simulink model "dcmg"  (R2020a)
settings: Solver=VariableStepAuto  StartTime=0.0  StopTime=Inf  FixedStep=50e-6  RelTol=1e-3
PostLoadFcn:
  | , if any(exist('dsrtsu_mdlpostloadfcn', 'file') ~= 0), dsrtsu_mdlpostloadfcn('Execute', bdroot); end,
InitFcn:
  | , if any(exist('rtifpga_mdlclblib', 'file') ~= 0), rtifpga_mdlclblib('Init', bdroot); end,
model workspace (MAT data in the model file):
  FPGA_dcmg_1_Register_1_1_1_write = Simulink.Signal
  FPGA_dcmg_1_Register_1_1_1_write.Description = 'RTIFPGA'
  FPGA_dcmg_1_Register_1_1_1_write.DataType = 'double'
  FPGA_dcmg_1_Register_1_1_1_write.Dimensions = '1'
  FPGA_dcmg_1_Register_1_1_1_write.DimensionsMode = 'auto'
  FPGA_dcmg_1_Register_1_1_1_write.Complexity = 'auto'
  FPGA_dcmg_1_Register_1_1_1_write.SampleTime = -1
  FPGA_dcmg_1_Register_1_1_1_write.SamplingMode = 'auto'
  FPGA_dcmg_1_Register_2_1_1_write = Simulink.Signal
  FPGA_dcmg_1_Register_2_1_1_write.Description = 'RTIFPGA'
  FPGA_dcmg_1_Register_2_1_1_write.DataType = 'double'
  FPGA_dcmg_1_Register_2_1_1_write.Dimensions = '1'
  FPGA_dcmg_1_Register_2_1_1_write.DimensionsMode = 'auto'
  FPGA_dcmg_1_Register_2_1_1_write.Complexity = 'auto'
  FPGA_dcmg_1_Register_2_1_1_write.SampleTime = -1
  FPGA_dcmg_1_Register_2_1_1_write.SamplingMode = 'auto'
  FPGA_dcmg_1_Register_3_1_1_write = Simulink.Signal
  FPGA_dcmg_1_Register_3_1_1_write.Description = 'RTIFPGA'
  FPGA_dcmg_1_Register_3_1_1_write.DataType = 'double'
  FPGA_dcmg_1_Register_3_1_1_write.Dimensions = '1'
  FPGA_dcmg_1_Register_3_1_1_write.DimensionsMode = 'auto'
  FPGA_dcmg_1_Register_3_1_1_write.Complexity = 'auto'
  FPGA_dcmg_1_Register_3_1_1_write.SampleTime = -1
  FPGA_dcmg_1_Register_3_1_1_write.SamplingMode = 'auto'
  FPGA_dcmg_1_Register_4_1_1_write = Simulink.Signal
  FPGA_dcmg_1_Register_4_1_1_write.Description = 'RTIFPGA'
  FPGA_dcmg_1_Register_4_1_1_write.DataType = 'double'
  FPGA_dcmg_1_Register_4_1_1_write.Dimensions = '1'
  FPGA_dcmg_1_Register_4_1_1_write.DimensionsMode = 'auto'
  FPGA_dcmg_1_Register_4_1_1_write.Complexity = 'auto'
  FPGA_dcmg_1_Register_4_1_1_write.SampleTime = -1
  FPGA_dcmg_1_Register_4_1_1_write.SamplingMode = 'auto'
  FPGA_dcmg_1_Register_5_1_1_write = Simulink.Signal
  FPGA_dcmg_1_Register_5_1_1_write.Description = 'RTIFPGA'
  FPGA_dcmg_1_Register_5_1_1_write.DataType = 'double'
  FPGA_dcmg_1_Register_5_1_1_write.Dimensions = '1'
  FPGA_dcmg_1_Register_5_1_1_write.DimensionsMode = 'auto'
  FPGA_dcmg_1_Register_5_1_1_write.Complexity = 'auto'
  FPGA_dcmg_1_Register_5_1_1_write.SampleTime = -1
  FPGA_dcmg_1_Register_5_1_1_write.SamplingMode = 'auto'
values from neighbouring files (symbols this model uses):
  den = [1, zeros(1,499)]    [params.m]
  fixedgain_i = 10*1000/(3*100)    (= 33.3333333333)    [param.m]    (also in params.m)
  fixedgain_ibat = 10*1000/(3*100)    (= 33.3333333333)    [params.m]
  fixedgain_ipv = 10*1000/(3*100)    (= 33.3333333333)    [params.m]
  fixedgain_v = 10*22000/(3*100*2.5)    (= 293.333333333)    [params.m]
  fixedgain_vdc = 10*22000/(3*100*2.5)    (= 293.333333333)    [param.m]    (also in params.m = 586.666666667)
  fixedgain_vpv = 10*10000/(3*100*2.5)    (= 133.333333333)    [params.m]
  gain_iavsi = 1    [params.m]
  gain_ibat = 1    [params.m]
  gain_ibvsi = 1    [params.m]
  gain_icvsi = 1    [params.m]
  gain_ioavsi = 1    [params.m]
  gain_iobvsi = 1    [params.m]
  gain_ipv = 1    [params.m]
  gain_sinwave = 0.3    [params.m]
  gain_vavsi = 1    [params.m]
  gain_vbvsi = 1    [params.m]
  gain_vcvsi = 1    [params.m]
  gain_vdc = 1    [param.m]    (also in params.m)
  gain_vpv = 1    [params.m]
  N = 10    [param.m]    (also in params.m = 100)
  num = 1/500*ones(1,500)    [params.m]
  offset_iavsi = 0.2    [params.m]
  offset_ibat = 0    [params.m]
  offset_ibvsi = 0.2    [params.m]
  offset_icvsi = 0.2    [params.m]
  offset_ioavsi = 0    [params.m]
  offset_iobvsi = 0    [params.m]
  offset_ipv = 0    [params.m]
  offset_vavsi = 0    [params.m]
  offset_vbvsi = 0    [params.m]
  offset_vcvsi = 0    [params.m]
  offset_vdc = 1.5    [param.m]    (also in params.m = 0)
  offset_vpv = 0    [params.m]
  v_dc_ref = 40    [param.m]    (also in params.m = 24)
libraries: xbsIndex_r4 x258, rti1202lib_adc_class1 x10, rtiproclib x9, simulink x5, rti1202lib_adc_class2 x2, rtifpgainterfacelib x1
(part 1 of 7)
Description:
  | Standard RTI1202 template.
  | Supported MATLAB version:  R2020a.
settings Model: Tag=RTI1202  DSRTSU_INTERNAL_RTI_VER=570  DSRTSU_INTERNAL_RTI_TYPE=rti1202  RTICANMMDATA=struct('GeneralSetupData',struct('modelroot','D:\MarcosGomez\DCMG','generalsettings',struct('filesettings',struct('destfolder',struct('Name','RTICANMM_FILES','Check',1),'buildfolder',struct('Name','.','Check',1),'AbsDestfolder',struct('Name','D:\MarcosGomez\DCMG\RTICANMM_FILES'),'AbsBuildfolder',struct('Name','D:\MarcosGomez\DCMG'))),'options',struct('addpaths',1,'rmpaths',1,'addtrcexclusion',true,'cannavigator',struct('checkmonitoring',0),'show_usrtrc',0,'use_usrtrc',0),'advanced',struct('options',ones(1,100)),'MPSetup',{{}},'RTI',struct('Type','RTI1202','Ver','7.15','Date','02-Nov-2020'),'modelname','dcmg','block','dcmg'))  DSRTSU_INTERNAL_RTIFPGA=170  OrderedModelArguments=off  Creator=dspace  LastModifiedBy=dspace
settings DataIOCC: ReturnWorkspaceOutputs=off
settings OptimizationCC: BlockReduction=off  OptimizeBlockIOStorage=off  BufferReuse=off  GlobalBufferReuse=off  ExpressionFolding=off  LocalBlockOutputs=off  OptimizeDataStoreBuffers=off  BusAssignmentInplaceUpdate=off
settings DebuggingCC: PregeneratedLibrarySubsystemCodeDiagnostic=none  ArithmeticOperatorsInVariantConditions=warning
settings HardwareCC: ProdBitPerPointer=32  ProdBitPerSizeT=32  ProdBitPerPtrDiffT=32  ProdLargestAtomicInteger=Integer  ProdEndianess=BigEndian  ProdWordSize=32  ProdLongLongMode=on  ProdHWDeviceType=Custom Processor->Custom  TargetIntDivRoundTo=Zero  TargetEndianess=BigEndian  TargetHWDeviceType=Custom Processor->Custom
settings ModelReferenceCC: EnableParallelModelReferenceBuilds=on  ParallelModelReferenceMATLABWorkerInit=Load Top Model
settings SFSimCC: SimUseLocalCustomCode=off  MATLABDynamicMemAlloc=off  CustomCodeUndefinedFunction=UseInterfaceOnly
settings RTWCC: Description=dSPACE DS1202 Hardware Platform  SystemTargetFile=rti1202.tlc  MakeCommand=make_rti  TemplateMakefile=rti1202.tmf  RTWUseLocalCustomCode=off
settings CodeAppCC: StateflowObjectComments=on
settings STFCustomTargetCC: ParMdlRefBuildCompliant=on  SystemTargetFile=rti1202.tlc
settings GRTTargetCC: TargetLangStandard=C89/C90 (ANSI)  CompOptLevelCompliant=off  ConcurrentExecutionCompliant=off  CombineOutputUpdateFcns=off  MatFileLogging=off  CPPClassGenCompliant=off  UseToolchainInfoCompliant=off
settings ConfigComp: CovMetricSettings=dswe

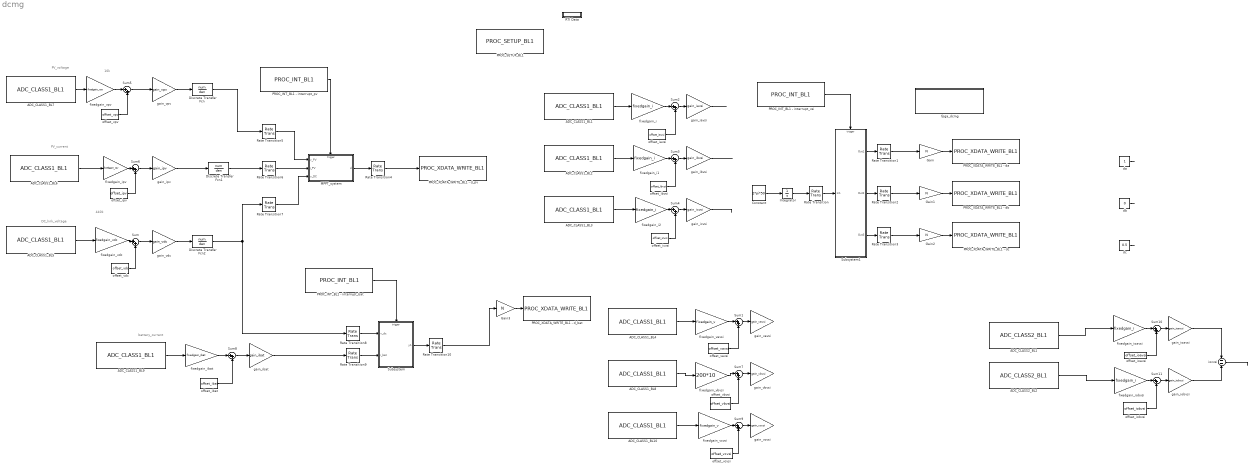
== system dcmg ==
  note: PV_voltage
  note: 10k
  note: 440k
  note: DC_link_voltage
  note: PV_current
  note: battery_current
  ADC_CLASS1_BL1 : rti1202lib_adc_class1/ADC_CLASS1_BL1  DSProperties=struct('RTI',struct('Version',uint32(1),'BlockType',struct('isSLSource',uint8(1),'isSLSink',uint8(1),'isHWSource',uint8(0),'isHWSink',uint8(1),'isSetup',uint8(0),'isInline',uint8(1),'isNonInline',uint8(0),'isInterrupt',uint8(0),'isChannelwise',uint8(1)),'IOBoardType',{{'DS120X','STD','ADCC1'}},'UnitType','ADC','Identifier','ADC','DialogType','ML','BlockSet','NONE','SlaveProcessor','NONE'))  RTIBlockInterface=struct('InputPortsActive',0,'InputPortsWidth',int32(1),'InputPortsDataType',{{'SS_BOOLEAN'}},'InputPortsName',{{'Continue'}},'OutputPortsActive',[1 0],'OutputPortsWidth',int32([1 1]),'OutputPortsDataType',{{'SS_DOUBLE','SS_INT16'}},'OutputPortsName',{{'ADC','Status'}},'DialogFcn','rti120xstdadcc1adcgui','SampleTime',{{-1}},'InitLevel',3,'IconTransparency','on','BlockDisplay',{{['ADC CL1\nChannel: 15'],'center'}},'BlockName',struct('Token',{{'ADC_CLASS1_BL1'}}))  RTIBlockParameters=struct('ReadMode',{{1,'OFF',[1 2]}},'ChannelNo',{{15,'OFF',[]}},'ConversionMode',{{1,'OFF',[1 2]}},'TriggerSource',{{1,'OFF',[1 2]}},'TriggerLineIn',{{1,'OFF',[1 16]}},'SampleMode',{{1,'OFF',[1 2]}},'BurstTriggerSource',{{1,'OFF',[1 2]}},'BurstTriggerLine',{{1,'OFF',[1 16]}},'ConvTriggerSource',{{3,'OFF',[1 3]}},'ConvTriggerLine',{{1,'OFF',[1 16]}},'ConvPeriod',{{'100e-6','OFF',[1e-6 1.34]}},'ConvPeriodCheck',{{0,'OFF',[]}},'BurstSize',{{'10','OFF',[]}},'BurstSizeCheck',{{0,'OFF',[]}},'DataSetOffset',{{'0','OFF',[]}},'DataSetOffsetCheck',{{0,'OFF',[]}},'DataSetLength',{{'1','OFF',[]}},'DataSetLengthCheck',{{0,'OFF',[]}},'EnableTriggerEvent',{{0,'OFF',[0 1]}},'TriggerMode',{{2,'OFF',[1 3]}},'TriggerLineOut',{{1,'OFF',[1 16]}},'ADCSWStartEnable',{{0,'OFF',[0 1]}},'SampleTime',{{'-1','OFF',[-1 inf]}},'SampleTimeCheck',{{1,'OFF',[]}},'StatusPortEnable',{{0,'OFF',[0 1]}},'TLCFileName',{{'rti120xadc_c1_adc','OFF',[]}})  RTISFcnParameters=struct('ReadMode','int16','ChannelNo','int16','ConversionMode','int16','TriggerSource','int16','TriggerLineIn','int16','SampleMode','int16','BurstTriggerSource','int16','BurstTriggerLine','int16','ConvTriggerSource','int16','ConvTriggerLine','int16','ConvPeriod','double','BurstSize','int16','DataSetOffset','int16','DataSetLength','int16','EnableTriggerEvent','int16','TriggerMode','int16','TriggerLineOut','int16','ADCSWStartEnable','int16','SampleTime','double','StatusPortEnable','int16','TLCFileName','char')  RTIBlockParaDefault=struct('ReadMode',1,'ChannelNo',1,'ConversionMode',1,'TriggerSource',1,'TriggerLineIn',1,'SampleMode',1,'BurstTriggerSource',1,'BurstTriggerLine',1,'ConvTriggerSource',3,'ConvTriggerLine',1,'ConvPeriod',0.0001,'ConvPeriodCheck',0,'BurstSize',10,'BurstSizeCheck',0,'DataSetOffset',0,'DataSetOffsetCheck',0,'DataSetLength',1,'DataSetLengthCheck',0,'EnableTriggerEvent',0,'TriggerMode',2,'TriggerLineOut',1,'ADCSWStartEnable',0,'SampleTime',-1,'SampleTimeCheck',1,'StatusPortEnable',0,'TLCFileName','rti120xadc_c1_adc')
  ADC_CLASS1_BL10 : rti1202lib_adc_class1/ADC_CLASS1_BL1  DSProperties=struct('RTI',struct('Version',uint32(1),'BlockType',struct('isSLSource',uint8(1),'isSLSink',uint8(1),'isHWSource',uint8(0),'isHWSink',uint8(1),'isSetup',uint8(0),'isInline',uint8(1),'isNonInline',uint8(0),'isInterrupt',uint8(0),'isChannelwise',uint8(1)),'IOBoardType',{{'DS120X','STD','ADCC1'}},'UnitType','ADC','Identifier','ADC','DialogType','ML','BlockSet','NONE','SlaveProcessor','NONE'))  RTIBlockInterface=struct('InputPortsActive',0,'InputPortsWidth',int32(1),'InputPortsDataType',{{'SS_BOOLEAN'}},'InputPortsName',{{'Continue'}},'OutputPortsActive',[1 0],'OutputPortsWidth',int32([1 1]),'OutputPortsDataType',{{'SS_DOUBLE','SS_INT16'}},'OutputPortsName',{{'ADC','Status'}},'DialogFcn','rti120xstdadcc1adcgui','SampleTime',{{-1}},'InitLevel',3,'IconTransparency','on','BlockDisplay',{{['ADC CL1\nChannel: 20'],'center'}},'BlockName',struct('Token',{{'ADC_CLASS1_BL1'}}))  RTIBlockParameters=struct('ReadMode',{{1,'OFF',[1 2]}},'ChannelNo',{{20,'OFF',[]}},'ConversionMode',{{1,'OFF',[1 2]}},'TriggerSource',{{1,'OFF',[1 2]}},'TriggerLineIn',{{1,'OFF',[1 16]}},'SampleMode',{{1,'OFF',[1 2]}},'BurstTriggerSource',{{1,'OFF',[1 2]}},'BurstTriggerLine',{{1,'OFF',[1 16]}},'ConvTriggerSource',{{3,'OFF',[1 3]}},'ConvTriggerLine',{{1,'OFF',[1 16]}},'ConvPeriod',{{'100e-6','OFF',[1e-6 1.34]}},'ConvPeriodCheck',{{0,'OFF',[]}},'BurstSize',{{'10','OFF',[]}},'BurstSizeCheck',{{0,'OFF',[]}},'DataSetOffset',{{'0','OFF',[]}},'DataSetOffsetCheck',{{0,'OFF',[]}},'DataSetLength',{{'1','OFF',[]}},'DataSetLengthCheck',{{0,'OFF',[]}},'EnableTriggerEvent',{{0,'OFF',[0 1]}},'TriggerMode',{{2,'OFF',[1 3]}},'TriggerLineOut',{{1,'OFF',[1 16]}},'ADCSWStartEnable',{{0,'OFF',[0 1]}},'SampleTime',{{'-1','OFF',[-1 inf]}},'SampleTimeCheck',{{1,'OFF',[]}},'StatusPortEnable',{{0,'OFF',[0 1]}},'TLCFileName',{{'rti120xadc_c1_adc','OFF',[]}})  RTISFcnParameters=struct('ReadMode','int16','ChannelNo','int16','ConversionMode','int16','TriggerSource','int16','TriggerLineIn','int16','SampleMode','int16','BurstTriggerSource','int16','BurstTriggerLine','int16','ConvTriggerSource','int16','ConvTriggerLine','int16','ConvPeriod','double','BurstSize','int16','DataSetOffset','int16','DataSetLength','int16','EnableTriggerEvent','int16','TriggerMode','int16','TriggerLineOut','int16','ADCSWStartEnable','int16','SampleTime','double','StatusPortEnable','int16','TLCFileName','char')  RTIBlockParaDefault=struct('ReadMode',1,'ChannelNo',1,'ConversionMode',1,'TriggerSource',1,'TriggerLineIn',1,'SampleMode',1,'BurstTriggerSource',1,'BurstTriggerLine',1,'ConvTriggerSource',3,'ConvTriggerLine',1,'ConvPeriod',0.0001,'ConvPeriodCheck',0,'BurstSize',10,'BurstSizeCheck',0,'DataSetOffset',0,'DataSetOffsetCheck',0,'DataSetLength',1,'DataSetLengthCheck',0,'EnableTriggerEvent',0,'TriggerMode',2,'TriggerLineOut',1,'ADCSWStartEnable',0,'SampleTime',-1,'SampleTimeCheck',1,'StatusPortEnable',0,'TLCFileName','rti120xadc_c1_adc')
  ADC_CLASS1_BL2 : rti1202lib_adc_class1/ADC_CLASS1_BL1  DSProperties=struct('RTI',struct('Version',uint32(1),'BlockType',struct('isSLSource',uint8(1),'isSLSink',uint8(1),'isHWSource',uint8(0),'isHWSink',uint8(1),'isSetup',uint8(0),'isInline',uint8(1),'isNonInline',uint8(0),'isInterrupt',uint8(0),'isChannelwise',uint8(1)),'IOBoardType',{{'DS120X','STD','ADCC1'}},'UnitType','ADC','Identifier','ADC','DialogType','ML','BlockSet','NONE','SlaveProcessor','NONE'))  RTIBlockInterface=struct('InputPortsActive',0,'InputPortsWidth',int32(1),'InputPortsDataType',{{'SS_BOOLEAN'}},'InputPortsName',{{'Continue'}},'OutputPortsActive',[1 0],'OutputPortsWidth',int32([1 1]),'OutputPortsDataType',{{'SS_DOUBLE','SS_INT16'}},'OutputPortsName',{{'ADC','Status'}},'DialogFcn','rti120xstdadcc1adcgui','SampleTime',{{-1}},'InitLevel',3,'IconTransparency','on','BlockDisplay',{{['ADC CL1\nChannel: 16'],'center'}},'BlockName',struct('Token',{{'ADC_CLASS1_BL1'}}))  RTIBlockParameters=struct('ReadMode',{{1,'OFF',[1 2]}},'ChannelNo',{{16,'OFF',[]}},'ConversionMode',{{1,'OFF',[1 2]}},'TriggerSource',{{1,'OFF',[1 2]}},'TriggerLineIn',{{1,'OFF',[1 16]}},'SampleMode',{{1,'OFF',[1 2]}},'BurstTriggerSource',{{1,'OFF',[1 2]}},'BurstTriggerLine',{{1,'OFF',[1 16]}},'ConvTriggerSource',{{3,'OFF',[1 3]}},'ConvTriggerLine',{{1,'OFF',[1 16]}},'ConvPeriod',{{'100e-6','OFF',[1e-6 1.34]}},'ConvPeriodCheck',{{0,'OFF',[]}},'BurstSize',{{'10','OFF',[]}},'BurstSizeCheck',{{0,'OFF',[]}},'DataSetOffset',{{'0','OFF',[]}},'DataSetOffsetCheck',{{0,'OFF',[]}},'DataSetLength',{{'1','OFF',[]}},'DataSetLengthCheck',{{0,'OFF',[]}},'EnableTriggerEvent',{{0,'OFF',[0 1]}},'TriggerMode',{{2,'OFF',[1 3]}},'TriggerLineOut',{{1,'OFF',[1 16]}},'ADCSWStartEnable',{{0,'OFF',[0 1]}},'SampleTime',{{'-1','OFF',[-1 inf]}},'SampleTimeCheck',{{1,'OFF',[]}},'StatusPortEnable',{{0,'OFF',[0 1]}},'TLCFileName',{{'rti120xadc_c1_adc','OFF',[]}})  RTISFcnParameters=struct('ReadMode','int16','ChannelNo','int16','ConversionMode','int16','TriggerSource','int16','TriggerLineIn','int16','SampleMode','int16','BurstTriggerSource','int16','BurstTriggerLine','int16','ConvTriggerSource','int16','ConvTriggerLine','int16','ConvPeriod','double','BurstSize','int16','DataSetOffset','int16','DataSetLength','int16','EnableTriggerEvent','int16','TriggerMode','int16','TriggerLineOut','int16','ADCSWStartEnable','int16','SampleTime','double','StatusPortEnable','int16','TLCFileName','char')  RTIBlockParaDefault=struct('ReadMode',1,'ChannelNo',1,'ConversionMode',1,'TriggerSource',1,'TriggerLineIn',1,'SampleMode',1,'BurstTriggerSource',1,'BurstTriggerLine',1,'ConvTriggerSource',3,'ConvTriggerLine',1,'ConvPeriod',0.0001,'ConvPeriodCheck',0,'BurstSize',10,'BurstSizeCheck',0,'DataSetOffset',0,'DataSetOffsetCheck',0,'DataSetLength',1,'DataSetLengthCheck',0,'EnableTriggerEvent',0,'TriggerMode',2,'TriggerLineOut',1,'ADCSWStartEnable',0,'SampleTime',-1,'SampleTimeCheck',1,'StatusPortEnable',0,'TLCFileName','rti120xadc_c1_adc')
  ADC_CLASS1_BL3 : rti1202lib_adc_class1/ADC_CLASS1_BL1  DSProperties=struct('RTI',struct('Version',uint32(1),'BlockType',struct('isSLSource',uint8(1),'isSLSink',uint8(1),'isHWSource',uint8(0),'isHWSink',uint8(1),'isSetup',uint8(0),'isInline',uint8(1),'isNonInline',uint8(0),'isInterrupt',uint8(0),'isChannelwise',uint8(1)),'IOBoardType',{{'DS120X','STD','ADCC1'}},'UnitType','ADC','Identifier','ADC','DialogType','ML','BlockSet','NONE','SlaveProcessor','NONE'))  RTIBlockInterface=struct('InputPortsActive',0,'InputPortsWidth',int32(1),'InputPortsDataType',{{'SS_BOOLEAN'}},'InputPortsName',{{'Continue'}},'OutputPortsActive',[1 0],'OutputPortsWidth',int32([1 1]),'OutputPortsDataType',{{'SS_DOUBLE','SS_INT16'}},'OutputPortsName',{{'ADC','Status'}},'DialogFcn','rti120xstdadcc1adcgui','SampleTime',{{-1}},'InitLevel',3,'IconTransparency','on','BlockDisplay',{{['ADC CL1\nChannel: 17'],'center'}},'BlockName',struct('Token',{{'ADC_CLASS1_BL1'}}))  RTIBlockParameters=struct('ReadMode',{{1,'OFF',[1 2]}},'ChannelNo',{{17,'OFF',[]}},'ConversionMode',{{1,'OFF',[1 2]}},'TriggerSource',{{1,'OFF',[1 2]}},'TriggerLineIn',{{1,'OFF',[1 16]}},'SampleMode',{{1,'OFF',[1 2]}},'BurstTriggerSource',{{1,'OFF',[1 2]}},'BurstTriggerLine',{{1,'OFF',[1 16]}},'ConvTriggerSource',{{3,'OFF',[1 3]}},'ConvTriggerLine',{{1,'OFF',[1 16]}},'ConvPeriod',{{'100e-6','OFF',[1e-6 1.34]}},'ConvPeriodCheck',{{0,'OFF',[]}},'BurstSize',{{'10','OFF',[]}},'BurstSizeCheck',{{0,'OFF',[]}},'DataSetOffset',{{'0','OFF',[]}},'DataSetOffsetCheck',{{0,'OFF',[]}},'DataSetLength',{{'1','OFF',[]}},'DataSetLengthCheck',{{0,'OFF',[]}},'EnableTriggerEvent',{{0,'OFF',[0 1]}},'TriggerMode',{{2,'OFF',[1 3]}},'TriggerLineOut',{{1,'OFF',[1 16]}},'ADCSWStartEnable',{{0,'OFF',[0 1]}},'SampleTime',{{'-1','OFF',[-1 inf]}},'SampleTimeCheck',{{1,'OFF',[]}},'StatusPortEnable',{{0,'OFF',[0 1]}},'TLCFileName',{{'rti120xadc_c1_adc','OFF',[]}})  RTISFcnParameters=struct('ReadMode','int16','ChannelNo','int16','ConversionMode','int16','TriggerSource','int16','TriggerLineIn','int16','SampleMode','int16','BurstTriggerSource','int16','BurstTriggerLine','int16','ConvTriggerSource','int16','ConvTriggerLine','int16','ConvPeriod','double','BurstSize','int16','DataSetOffset','int16','DataSetLength','int16','EnableTriggerEvent','int16','TriggerMode','int16','TriggerLineOut','int16','ADCSWStartEnable','int16','SampleTime','double','StatusPortEnable','int16','TLCFileName','char')  RTIBlockParaDefault=struct('ReadMode',1,'ChannelNo',1,'ConversionMode',1,'TriggerSource',1,'TriggerLineIn',1,'SampleMode',1,'BurstTriggerSource',1,'BurstTriggerLine',1,'ConvTriggerSource',3,'ConvTriggerLine',1,'ConvPeriod',0.0001,'ConvPeriodCheck',0,'BurstSize',10,'BurstSizeCheck',0,'DataSetOffset',0,'DataSetOffsetCheck',0,'DataSetLength',1,'DataSetLengthCheck',0,'EnableTriggerEvent',0,'TriggerMode',2,'TriggerLineOut',1,'ADCSWStartEnable',0,'SampleTime',-1,'SampleTimeCheck',1,'StatusPortEnable',0,'TLCFileName','rti120xadc_c1_adc')
  ADC_CLASS1_BL4 : rti1202lib_adc_class1/ADC_CLASS1_BL1  DSProperties=struct('RTI',struct('Version',uint32(1),'BlockType',struct('isSLSource',uint8(1),'isSLSink',uint8(1),'isHWSource',uint8(0),'isHWSink',uint8(1),'isSetup',uint8(0),'isInline',uint8(1),'isNonInline',uint8(0),'isInterrupt',uint8(0),'isChannelwise',uint8(1)),'IOBoardType',{{'DS120X','STD','ADCC1'}},'UnitType','ADC','Identifier','ADC','DialogType','ML','BlockSet','NONE','SlaveProcessor','NONE'))  RTIBlockInterface=struct('InputPortsActive',0,'InputPortsWidth',int32(1),'InputPortsDataType',{{'SS_BOOLEAN'}},'InputPortsName',{{'Continue'}},'OutputPortsActive',[1 0],'OutputPortsWidth',int32([1 1]),'OutputPortsDataType',{{'SS_DOUBLE','SS_INT16'}},'OutputPortsName',{{'ADC','Status'}},'DialogFcn','rti120xstdadcc1adcgui','SampleTime',{{-1}},'InitLevel',3,'IconTransparency','on','BlockDisplay',{{['ADC CL1\nChannel: 18'],'center'}},'BlockName',struct('Token',{{'ADC_CLASS1_BL1'}}))  RTIBlockParameters=struct('ReadMode',{{1,'OFF',[1 2]}},'ChannelNo',{{18,'OFF',[]}},'ConversionMode',{{1,'OFF',[1 2]}},'TriggerSource',{{1,'OFF',[1 2]}},'TriggerLineIn',{{1,'OFF',[1 16]}},'SampleMode',{{1,'OFF',[1 2]}},'BurstTriggerSource',{{1,'OFF',[1 2]}},'BurstTriggerLine',{{1,'OFF',[1 16]}},'ConvTriggerSource',{{3,'OFF',[1 3]}},'ConvTriggerLine',{{1,'OFF',[1 16]}},'ConvPeriod',{{'100e-6','OFF',[1e-6 1.34]}},'ConvPeriodCheck',{{0,'OFF',[]}},'BurstSize',{{'10','OFF',[]}},'BurstSizeCheck',{{0,'OFF',[]}},'DataSetOffset',{{'0','OFF',[]}},'DataSetOffsetCheck',{{0,'OFF',[]}},'DataSetLength',{{'1','OFF',[]}},'DataSetLengthCheck',{{0,'OFF',[]}},'EnableTriggerEvent',{{0,'OFF',[0 1]}},'TriggerMode',{{2,'OFF',[1 3]}},'TriggerLineOut',{{1,'OFF',[1 16]}},'ADCSWStartEnable',{{0,'OFF',[0 1]}},'SampleTime',{{'-1','OFF',[-1 inf]}},'SampleTimeCheck',{{1,'OFF',[]}},'StatusPortEnable',{{0,'OFF',[0 1]}},'TLCFileName',{{'rti120xadc_c1_adc','OFF',[]}})  RTISFcnParameters=struct('ReadMode','int16','ChannelNo','int16','ConversionMode','int16','TriggerSource','int16','TriggerLineIn','int16','SampleMode','int16','BurstTriggerSource','int16','BurstTriggerLine','int16','ConvTriggerSource','int16','ConvTriggerLine','int16','ConvPeriod','double','BurstSize','int16','DataSetOffset','int16','DataSetLength','int16','EnableTriggerEvent','int16','TriggerMode','int16','TriggerLineOut','int16','ADCSWStartEnable','int16','SampleTime','double','StatusPortEnable','int16','TLCFileName','char')  RTIBlockParaDefault=struct('ReadMode',1,'ChannelNo',1,'ConversionMode',1,'TriggerSource',1,'TriggerLineIn',1,'SampleMode',1,'BurstTriggerSource',1,'BurstTriggerLine',1,'ConvTriggerSource',3,'ConvTriggerLine',1,'ConvPeriod',0.0001,'ConvPeriodCheck',0,'BurstSize',10,'BurstSizeCheck',0,'DataSetOffset',0,'DataSetOffsetCheck',0,'DataSetLength',1,'DataSetLengthCheck',0,'EnableTriggerEvent',0,'TriggerMode',2,'TriggerLineOut',1,'ADCSWStartEnable',0,'SampleTime',-1,'SampleTimeCheck',1,'StatusPortEnable',0,'TLCFileName','rti120xadc_c1_adc')
  ADC_CLASS1_BL5 : rti1202lib_adc_class1/ADC_CLASS1_BL1  DSProperties=struct('RTI',struct('Version',uint32(1),'BlockType',struct('isSLSource',uint8(1),'isSLSink',uint8(1),'isHWSource',uint8(0),'isHWSink',uint8(1),'isSetup',uint8(0),'isInline',uint8(1),'isNonInline',uint8(0),'isInterrupt',uint8(0),'isChannelwise',uint8(1)),'IOBoardType',{{'DS120X','STD','ADCC1'}},'UnitType','ADC','Identifier','ADC','DialogType','ML','BlockSet','NONE','SlaveProcessor','NONE'))  RTIBlockInterface=struct('InputPortsActive',0,'InputPortsWidth',int32(1),'InputPortsDataType',{{'SS_BOOLEAN'}},'InputPortsName',{{'Continue'}},'OutputPortsActive',[1 0],'OutputPortsWidth',int32([1 1]),'OutputPortsDataType',{{'SS_DOUBLE','SS_INT16'}},'OutputPortsName',{{'ADC','Status'}},'DialogFcn','rti120xstdadcc1adcgui','SampleTime',{{-1}},'InitLevel',3,'IconTransparency','on','BlockDisplay',{{['ADC CL1\nChannel: 24'],'center'}},'BlockName',struct('Token',{{'ADC_CLASS1_BL1'}}))  RTIBlockParameters=struct('ReadMode',{{1,'OFF',[1 2]}},'ChannelNo',{{24,'OFF',[]}},'ConversionMode',{{1,'OFF',[1 2]}},'TriggerSource',{{1,'OFF',[1 2]}},'TriggerLineIn',{{1,'OFF',[1 16]}},'SampleMode',{{1,'OFF',[1 2]}},'BurstTriggerSource',{{1,'OFF',[1 2]}},'BurstTriggerLine',{{1,'OFF',[1 16]}},'ConvTriggerSource',{{3,'OFF',[1 3]}},'ConvTriggerLine',{{1,'OFF',[1 16]}},'ConvPeriod',{{'100e-6','OFF',[1e-6 1.34]}},'ConvPeriodCheck',{{0,'OFF',[]}},'BurstSize',{{'10','OFF',[]}},'BurstSizeCheck',{{0,'OFF',[]}},'DataSetOffset',{{'0','OFF',[]}},'DataSetOffsetCheck',{{0,'OFF',[]}},'DataSetLength',{{'1','OFF',[]}},'DataSetLengthCheck',{{0,'OFF',[]}},'EnableTriggerEvent',{{0,'OFF',[0 1]}},'TriggerMode',{{2,'OFF',[1 3]}},'TriggerLineOut',{{1,'OFF',[1 16]}},'ADCSWStartEnable',{{0,'OFF',[0 1]}},'SampleTime',{{'-1','OFF',[-1 inf]}},'SampleTimeCheck',{{1,'OFF',[]}},'StatusPortEnable',{{0,'OFF',[0 1]}},'TLCFileName',{{'rti120xadc_c1_adc','OFF',[]}})  RTISFcnParameters=struct('ReadMode','int16','ChannelNo','int16','ConversionMode','int16','TriggerSource','int16','TriggerLineIn','int16','SampleMode','int16','BurstTriggerSource','int16','BurstTriggerLine','int16','ConvTriggerSource','int16','ConvTriggerLine','int16','ConvPeriod','double','BurstSize','int16','DataSetOffset','int16','DataSetLength','int16','EnableTriggerEvent','int16','TriggerMode','int16','TriggerLineOut','int16','ADCSWStartEnable','int16','SampleTime','double','StatusPortEnable','int16','TLCFileName','char')  RTIBlockParaDefault=struct('ReadMode',1,'ChannelNo',1,'ConversionMode',1,'TriggerSource',1,'TriggerLineIn',1,'SampleMode',1,'BurstTriggerSource',1,'BurstTriggerLine',1,'ConvTriggerSource',3,'ConvTriggerLine',1,'ConvPeriod',0.0001,'ConvPeriodCheck',0,'BurstSize',10,'BurstSizeCheck',0,'DataSetOffset',0,'DataSetOffsetCheck',0,'DataSetLength',1,'DataSetLengthCheck',0,'EnableTriggerEvent',0,'TriggerMode',2,'TriggerLineOut',1,'ADCSWStartEnable',0,'SampleTime',-1,'SampleTimeCheck',1,'StatusPortEnable',0,'TLCFileName','rti120xadc_c1_adc')
  ADC_CLASS1_BL6 : rti1202lib_adc_class1/ADC_CLASS1_BL1  DSProperties=struct('RTI',struct('Version',uint32(1),'BlockType',struct('isSLSource',uint8(1),'isSLSink',uint8(1),'isHWSource',uint8(0),'isHWSink',uint8(1),'isSetup',uint8(0),'isInline',uint8(1),'isNonInline',uint8(0),'isInterrupt',uint8(0),'isChannelwise',uint8(1)),'IOBoardType',{{'DS120X','STD','ADCC1'}},'UnitType','ADC','Identifier','ADC','DialogType','ML','BlockSet','NONE','SlaveProcessor','NONE'))  RTIBlockInterface=struct('InputPortsActive',0,'InputPortsWidth',int32(1),'InputPortsDataType',{{'SS_BOOLEAN'}},'InputPortsName',{{'Continue'}},'OutputPortsActive',[1 0],'OutputPortsWidth',int32([1 1]),'OutputPortsDataType',{{'SS_DOUBLE','SS_INT16'}},'OutputPortsName',{{'ADC','Status'}},'DialogFcn','rti120xstdadcc1adcgui','SampleTime',{{-1}},'InitLevel',3,'IconTransparency','on','BlockDisplay',{{['ADC CL1\nChannel: 23'],'center'}},'BlockName',struct('Token',{{'ADC_CLASS1_BL1'}}))  RTIBlockParameters=struct('ReadMode',{{1,'OFF',[1 2]}},'ChannelNo',{{23,'OFF',[]}},'ConversionMode',{{1,'OFF',[1 2]}},'TriggerSource',{{1,'OFF',[1 2]}},'TriggerLineIn',{{1,'OFF',[1 16]}},'SampleMode',{{1,'OFF',[1 2]}},'BurstTriggerSource',{{1,'OFF',[1 2]}},'BurstTriggerLine',{{1,'OFF',[1 16]}},'ConvTriggerSource',{{3,'OFF',[1 3]}},'ConvTriggerLine',{{1,'OFF',[1 16]}},'ConvPeriod',{{'100e-6','OFF',[1e-6 1.34]}},'ConvPeriodCheck',{{0,'OFF',[]}},'BurstSize',{{'10','OFF',[]}},'BurstSizeCheck',{{0,'OFF',[]}},'DataSetOffset',{{'0','OFF',[]}},'DataSetOffsetCheck',{{0,'OFF',[]}},'DataSetLength',{{'1','OFF',[]}},'DataSetLengthCheck',{{0,'OFF',[]}},'EnableTriggerEvent',{{0,'OFF',[0 1]}},'TriggerMode',{{2,'OFF',[1 3]}},'TriggerLineOut',{{1,'OFF',[1 16]}},'ADCSWStartEnable',{{0,'OFF',[0 1]}},'SampleTime',{{'-1','OFF',[-1 inf]}},'SampleTimeCheck',{{1,'OFF',[]}},'StatusPortEnable',{{0,'OFF',[0 1]}},'TLCFileName',{{'rti120xadc_c1_adc','OFF',[]}})  RTISFcnParameters=struct('ReadMode','int16','ChannelNo','int16','ConversionMode','int16','TriggerSource','int16','TriggerLineIn','int16','SampleMode','int16','BurstTriggerSource','int16','BurstTriggerLine','int16','ConvTriggerSource','int16','ConvTriggerLine','int16','ConvPeriod','double','BurstSize','int16','DataSetOffset','int16','DataSetLength','int16','EnableTriggerEvent','int16','TriggerMode','int16','TriggerLineOut','int16','ADCSWStartEnable','int16','SampleTime','double','StatusPortEnable','int16','TLCFileName','char')  RTIBlockParaDefault=struct('ReadMode',1,'ChannelNo',1,'ConversionMode',1,'TriggerSource',1,'TriggerLineIn',1,'SampleMode',1,'BurstTriggerSource',1,'BurstTriggerLine',1,'ConvTriggerSource',3,'ConvTriggerLine',1,'ConvPeriod',0.0001,'ConvPeriodCheck',0,'BurstSize',10,'BurstSizeCheck',0,'DataSetOffset',0,'DataSetOffsetCheck',0,'DataSetLength',1,'DataSetLengthCheck',0,'EnableTriggerEvent',0,'TriggerMode',2,'TriggerLineOut',1,'ADCSWStartEnable',0,'SampleTime',-1,'SampleTimeCheck',1,'StatusPortEnable',0,'TLCFileName','rti120xadc_c1_adc')
  ADC_CLASS1_BL7 : rti1202lib_adc_class1/ADC_CLASS1_BL1  DSProperties=struct('RTI',struct('Version',uint32(1),'BlockType',struct('isSLSource',uint8(1),'isSLSink',uint8(1),'isHWSource',uint8(0),'isHWSink',uint8(1),'isSetup',uint8(0),'isInline',uint8(1),'isNonInline',uint8(0),'isInterrupt',uint8(0),'isChannelwise',uint8(1)),'IOBoardType',{{'DS120X','STD','ADCC1'}},'UnitType','ADC','Identifier','ADC','DialogType','ML','BlockSet','NONE','SlaveProcessor','NONE'))  RTIBlockInterface=struct('InputPortsActive',0,'InputPortsWidth',int32(1),'InputPortsDataType',{{'SS_BOOLEAN'}},'InputPortsName',{{'Continue'}},'OutputPortsActive',[1 0],'OutputPortsWidth',int32([1 1]),'OutputPortsDataType',{{'SS_DOUBLE','SS_INT16'}},'OutputPortsName',{{'ADC','Status'}},'DialogFcn','rti120xstdadcc1adcgui','SampleTime',{{-1}},'InitLevel',3,'IconTransparency','on','BlockDisplay',{{['ADC CL1\nChannel: 22'],'center'}},'BlockName',struct('Token',{{'ADC_CLASS1_BL1'}}))  RTIBlockParameters=struct('ReadMode',{{1,'OFF',[1 2]}},'ChannelNo',{{22,'OFF',[]}},'ConversionMode',{{1,'OFF',[1 2]}},'TriggerSource',{{1,'OFF',[1 2]}},'TriggerLineIn',{{1,'OFF',[1 16]}},'SampleMode',{{1,'OFF',[1 2]}},'BurstTriggerSource',{{1,'OFF',[1 2]}},'BurstTriggerLine',{{1,'OFF',[1 16]}},'ConvTriggerSource',{{3,'OFF',[1 3]}},'ConvTriggerLine',{{1,'OFF',[1 16]}},'ConvPeriod',{{'100e-6','OFF',[1e-6 1.34]}},'ConvPeriodCheck',{{0,'OFF',[]}},'BurstSize',{{'10','OFF',[]}},'BurstSizeCheck',{{0,'OFF',[]}},'DataSetOffset',{{'0','OFF',[]}},'DataSetOffsetCheck',{{0,'OFF',[]}},'DataSetLength',{{'1','OFF',[]}},'DataSetLengthCheck',{{0,'OFF',[]}},'EnableTriggerEvent',{{0,'OFF',[0 1]}},'TriggerMode',{{2,'OFF',[1 3]}},'TriggerLineOut',{{1,'OFF',[1 16]}},'ADCSWStartEnable',{{0,'OFF',[0 1]}},'SampleTime',{{'-1','OFF',[-1 inf]}},'SampleTimeCheck',{{1,'OFF',[]}},'StatusPortEnable',{{0,'OFF',[0 1]}},'TLCFileName',{{'rti120xadc_c1_adc','OFF',[]}})  RTISFcnParameters=struct('ReadMode','int16','ChannelNo','int16','ConversionMode','int16','TriggerSource','int16','TriggerLineIn','int16','SampleMode','int16','BurstTriggerSource','int16','BurstTriggerLine','int16','ConvTriggerSource','int16','ConvTriggerLine','int16','ConvPeriod','double','BurstSize','int16','DataSetOffset','int16','DataSetLength','int16','EnableTriggerEvent','int16','TriggerMode','int16','TriggerLineOut','int16','ADCSWStartEnable','int16','SampleTime','double','StatusPortEnable','int16','TLCFileName','char')  RTIBlockParaDefault=struct('ReadMode',1,'ChannelNo',1,'ConversionMode',1,'TriggerSource',1,'TriggerLineIn',1,'SampleMode',1,'BurstTriggerSource',1,'BurstTriggerLine',1,'ConvTriggerSource',3,'ConvTriggerLine',1,'ConvPeriod',0.0001,'ConvPeriodCheck',0,'BurstSize',10,'BurstSizeCheck',0,'DataSetOffset',0,'DataSetOffsetCheck',0,'DataSetLength',1,'DataSetLengthCheck',0,'EnableTriggerEvent',0,'TriggerMode',2,'TriggerLineOut',1,'ADCSWStartEnable',0,'SampleTime',-1,'SampleTimeCheck',1,'StatusPortEnable',0,'TLCFileName','rti120xadc_c1_adc')
  ADC_CLASS1_BL8 : rti1202lib_adc_class1/ADC_CLASS1_BL1  DSProperties=struct('RTI',struct('Version',uint32(1),'BlockType',struct('isSLSource',uint8(1),'isSLSink',uint8(1),'isHWSource',uint8(0),'isHWSink',uint8(1),'isSetup',uint8(0),'isInline',uint8(1),'isNonInline',uint8(0),'isInterrupt',uint8(0),'isChannelwise',uint8(1)),'IOBoardType',{{'DS120X','STD','ADCC1'}},'UnitType','ADC','Identifier','ADC','DialogType','ML','BlockSet','NONE','SlaveProcessor','NONE'))  RTIBlockInterface=struct('InputPortsActive',0,'InputPortsWidth',int32(1),'InputPortsDataType',{{'SS_BOOLEAN'}},'InputPortsName',{{'Continue'}},'OutputPortsActive',[1 0],'OutputPortsWidth',int32([1 1]),'OutputPortsDataType',{{'SS_DOUBLE','SS_INT16'}},'OutputPortsName',{{'ADC','Status'}},'DialogFcn','rti120xstdadcc1adcgui','SampleTime',{{-1}},'InitLevel',3,'IconTransparency','on','BlockDisplay',{{['ADC CL1\nChannel: 19'],'center'}},'BlockName',struct('Token',{{'ADC_CLASS1_BL1'}}))  RTIBlockParameters=struct('ReadMode',{{1,'OFF',[1 2]}},'ChannelNo',{{19,'OFF',[]}},'ConversionMode',{{1,'OFF',[1 2]}},'TriggerSource',{{1,'OFF',[1 2]}},'TriggerLineIn',{{1,'OFF',[1 16]}},'SampleMode',{{1,'OFF',[1 2]}},'BurstTriggerSource',{{1,'OFF',[1 2]}},'BurstTriggerLine',{{1,'OFF',[1 16]}},'ConvTriggerSource',{{3,'OFF',[1 3]}},'ConvTriggerLine',{{1,'OFF',[1 16]}},'ConvPeriod',{{'100e-6','OFF',[1e-6 1.34]}},'ConvPeriodCheck',{{0,'OFF',[]}},'BurstSize',{{'10','OFF',[]}},'BurstSizeCheck',{{0,'OFF',[]}},'DataSetOffset',{{'0','OFF',[]}},'DataSetOffsetCheck',{{0,'OFF',[]}},'DataSetLength',{{'1','OFF',[]}},'DataSetLengthCheck',{{0,'OFF',[]}},'EnableTriggerEvent',{{0,'OFF',[0 1]}},'TriggerMode',{{2,'OFF',[1 3]}},'TriggerLineOut',{{1,'OFF',[1 16]}},'ADCSWStartEnable',{{0,'OFF',[0 1]}},'SampleTime',{{'-1','OFF',[-1 inf]}},'SampleTimeCheck',{{1,'OFF',[]}},'StatusPortEnable',{{0,'OFF',[0 1]}},'TLCFileName',{{'rti120xadc_c1_adc','OFF',[]}})  RTISFcnParameters=struct('ReadMode','int16','ChannelNo','int16','ConversionMode','int16','TriggerSource','int16','TriggerLineIn','int16','SampleMode','int16','BurstTriggerSource','int16','BurstTriggerLine','int16','ConvTriggerSource','int16','ConvTriggerLine','int16','ConvPeriod','double','BurstSize','int16','DataSetOffset','int16','DataSetLength','int16','EnableTriggerEvent','int16','TriggerMode','int16','TriggerLineOut','int16','ADCSWStartEnable','int16','SampleTime','double','StatusPortEnable','int16','TLCFileName','char')  RTIBlockParaDefault=struct('ReadMode',1,'ChannelNo',1,'ConversionMode',1,'TriggerSource',1,'TriggerLineIn',1,'SampleMode',1,'BurstTriggerSource',1,'BurstTriggerLine',1,'ConvTriggerSource',3,'ConvTriggerLine',1,'ConvPeriod',0.0001,'ConvPeriodCheck',0,'BurstSize',10,'BurstSizeCheck',0,'DataSetOffset',0,'DataSetOffsetCheck',0,'DataSetLength',1,'DataSetLengthCheck',0,'EnableTriggerEvent',0,'TriggerMode',2,'TriggerLineOut',1,'ADCSWStartEnable',0,'SampleTime',-1,'SampleTimeCheck',1,'StatusPortEnable',0,'TLCFileName','rti120xadc_c1_adc')
  ADC_CLASS1_BL9 : rti1202lib_adc_class1/ADC_CLASS1_BL1  DSProperties=struct('RTI',struct('Version',uint32(1),'BlockType',struct('isSLSource',uint8(1),'isSLSink',uint8(1),'isHWSource',uint8(0),'isHWSink',uint8(1),'isSetup',uint8(0),'isInline',uint8(1),'isNonInline',uint8(0),'isInterrupt',uint8(0),'isChannelwise',uint8(1)),'IOBoardType',{{'DS120X','STD','ADCC1'}},'UnitType','ADC','Identifier','ADC','DialogType','ML','BlockSet','NONE','SlaveProcessor','NONE'))  RTIBlockInterface=struct('InputPortsActive',0,'InputPortsWidth',int32(1),'InputPortsDataType',{{'SS_BOOLEAN'}},'InputPortsName',{{'Continue'}},'OutputPortsActive',[1 0],'OutputPortsWidth',int32([1 1]),'OutputPortsDataType',{{'SS_DOUBLE','SS_INT16'}},'OutputPortsName',{{'ADC','Status'}},'DialogFcn','rti120xstdadcc1adcgui','SampleTime',{{-1}},'InitLevel',3,'IconTransparency','on','BlockDisplay',{{['ADC CL1\nChannel: 21'],'center'}},'BlockName',struct('Token',{{'ADC_CLASS1_BL1'}}))  RTIBlockParameters=struct('ReadMode',{{1,'OFF',[1 2]}},'ChannelNo',{{21,'OFF',[]}},'ConversionMode',{{1,'OFF',[1 2]}},'TriggerSource',{{1,'OFF',[1 2]}},'TriggerLineIn',{{1,'OFF',[1 16]}},'SampleMode',{{1,'OFF',[1 2]}},'BurstTriggerSource',{{1,'OFF',[1 2]}},'BurstTriggerLine',{{1,'OFF',[1 16]}},'ConvTriggerSource',{{3,'OFF',[1 3]}},'ConvTriggerLine',{{1,'OFF',[1 16]}},'ConvPeriod',{{'100e-6','OFF',[1e-6 1.34]}},'ConvPeriodCheck',{{0,'OFF',[]}},'BurstSize',{{'10','OFF',[]}},'BurstSizeCheck',{{0,'OFF',[]}},'DataSetOffset',{{'0','OFF',[]}},'DataSetOffsetCheck',{{0,'OFF',[]}},'DataSetLength',{{'1','OFF',[]}},'DataSetLengthCheck',{{0,'OFF',[]}},'EnableTriggerEvent',{{0,'OFF',[0 1]}},'TriggerMode',{{2,'OFF',[1 3]}},'TriggerLineOut',{{1,'OFF',[1 16]}},'ADCSWStartEnable',{{0,'OFF',[0 1]}},'SampleTime',{{'-1','OFF',[-1 inf]}},'SampleTimeCheck',{{1,'OFF',[]}},'StatusPortEnable',{{0,'OFF',[0 1]}},'TLCFileName',{{'rti120xadc_c1_adc','OFF',[]}})  RTISFcnParameters=struct('ReadMode','int16','ChannelNo','int16','ConversionMode','int16','TriggerSource','int16','TriggerLineIn','int16','SampleMode','int16','BurstTriggerSource','int16','BurstTriggerLine','int16','ConvTriggerSource','int16','ConvTriggerLine','int16','ConvPeriod','double','BurstSize','int16','DataSetOffset','int16','DataSetLength','int16','EnableTriggerEvent','int16','TriggerMode','int16','TriggerLineOut','int16','ADCSWStartEnable','int16','SampleTime','double','StatusPortEnable','int16','TLCFileName','char')  RTIBlockParaDefault=struct('ReadMode',1,'ChannelNo',1,'ConversionMode',1,'TriggerSource',1,'TriggerLineIn',1,'SampleMode',1,'BurstTriggerSource',1,'BurstTriggerLine',1,'ConvTriggerSource',3,'ConvTriggerLine',1,'ConvPeriod',0.0001,'ConvPeriodCheck',0,'BurstSize',10,'BurstSizeCheck',0,'DataSetOffset',0,'DataSetOffsetCheck',0,'DataSetLength',1,'DataSetLengthCheck',0,'EnableTriggerEvent',0,'TriggerMode',2,'TriggerLineOut',1,'ADCSWStartEnable',0,'SampleTime',-1,'SampleTimeCheck',1,'StatusPortEnable',0,'TLCFileName','rti120xadc_c1_adc')
  ADC_CLASS2_BL1 : rti1202lib_adc_class2/ADC_CLASS2_BL1  DSProperties=struct('RTI',struct('Version',uint32(1),'BlockType',struct('isSLSource',uint8(1),'isSLSink',uint8(1),'isHWSource',uint8(0),'isHWSink',uint8(1),'isSetup',uint8(0),'isInline',uint8(1),'isNonInline',uint8(0),'isInterrupt',uint8(0),'isChannelwise',uint8(1)),'IOBoardType',{{'DS120X','STD','ADCC2'}},'UnitType','ADC','Identifier','ADC','DialogType','ML','BlockSet','NONE','SlaveProcessor','NONE'))  RTIBlockInterface=struct('OutputPortsActive',1,'OutputPortsWidth',int32(1),'OutputPortsDataType',{{'SS_DOUBLE'}},'OutputPortsName',{{'ADC'}},'DialogFcn','rti120xstdadcc2adcgui','InitLevel',3,'IconTransparency','on','BlockDisplay',{{['ADC CL2\nChannel: 1'],'center'}},'BlockName',struct('Token',{{'ADC_CLASS2_BL1'}}))  RTIBlockParameters=struct('ChannelNo',{{1,'OFF',[]}},'TLCFileName',{{'rti120xadc_c2_adc','OFF',[]}})  RTISFcnParameters=struct('ChannelNo','int16','TLCFileName','char')  RTIBlockParaDefault=struct('ChannelNo',1,'TLCFileName','rti120xadc_c2_adc')
  ADC_CLASS2_BL2 : rti1202lib_adc_class2/ADC_CLASS2_BL1  DSProperties=struct('RTI',struct('Version',uint32(1),'BlockType',struct('isSLSource',uint8(1),'isSLSink',uint8(1),'isHWSource',uint8(0),'isHWSink',uint8(1),'isSetup',uint8(0),'isInline',uint8(1),'isNonInline',uint8(0),'isInterrupt',uint8(0),'isChannelwise',uint8(1)),'IOBoardType',{{'DS120X','STD','ADCC2'}},'UnitType','ADC','Identifier','ADC','DialogType','ML','BlockSet','NONE','SlaveProcessor','NONE'))  RTIBlockInterface=struct('OutputPortsActive',1,'OutputPortsWidth',int32(1),'OutputPortsDataType',{{'SS_DOUBLE'}},'OutputPortsName',{{'ADC'}},'DialogFcn','rti120xstdadcc2adcgui','InitLevel',3,'IconTransparency','on','BlockDisplay',{{['ADC CL2\nChannel: 2'],'center'}},'BlockName',struct('Token',{{'ADC_CLASS2_BL1'}}))  RTIBlockParameters=struct('ChannelNo',{{2,'OFF',[]}},'TLCFileName',{{'rti120xadc_c2_adc','OFF',[]}})  RTISFcnParameters=struct('ChannelNo','int16','TLCFileName','char')  RTIBlockParaDefault=struct('ChannelNo',1,'TLCFileName','rti120xadc_c2_adc')
  Constant : Constant  Value=2*pi*50
  Discrete Transfer Fcn : DiscreteTransferFcn  Numerator=num  Denominator=den
  Discrete Transfer Fcn1 : DiscreteTransferFcn  Numerator=num  Denominator=den
  Discrete Transfer Fcn2 : DiscreteTransferFcn  Numerator=num  Denominator=den
  Gain{,1..3} (4 alike) : Gain  Gain=N  OutMin=1  OutMax=999
  Integrator : Integrator
  MPPT_system : Subsystem
  PROC_INT_BL1 - interrupt_bat : rtiproclib/PROC_INT_BL1  DSProperties=struct('RTI',struct('Version',uint32(4),'BlockType',struct('isSLSource',uint8(1),'isSLSink',uint8(0),'isHWSource',uint8(0),'isHWSink',uint8(0),'isSetup',uint8(1),'isInline',uint8(1),'isNonInline',uint8(0),'isInterrupt',uint8(0),'isChannelwise',uint8(0)),'IOBoardType','DSPROC','UnitType','','Identifier','INT','DialogType','ML','BlockSet','DSPROC','SlaveProcessor',''))  RTIBlockInterface=struct('OutputPortsActive',1,'OutputPortsWidth',int32(1),'OutputPortsName',{{'Interrupt'}},'FunctionCall',uint32(0),'DialogFcn','rtiprocintgui','InitLevel',3,'BlockDisplay',{{['Interrupt In 2\ninterrupt_bat \nBoard: 1'],'center'}},'IconTransparency','on','BlockName',struct('Token',{{'PROC_INT_BL1'}}))  RTIBlockParameters=struct('BoardNo',{{'1','OFF',[1 16]}},'ChannelNo',{{'2','OFF',[1 8]}},'AccessTyp',{{'Interrupt','OFF',[]}},'BinaryPoint',{{'0','OFF',[]}},'DataFormat',{{'unsigned','OFF',[]}},'BufferLength',{{'0','OFF',[]}},'MultiChAccess',{{'0','OFF',[]}},'ModelPortBlock',{{{struct('BlockId','','SignalId','')},'OFF',[]}})  RTISFcnParameters=struct('BoardNo','double','ChannelNo','double','AccessTyp','char','BinaryPoint','double','DataFormat','char','BufferLength','double')  RTIBlockParaDefault=struct('BoardNo','1','ChannelNo','1','AccessTyp','Interrupt','BinaryPoint','10','DataFormat','unsigned','BufferLength','0','MultiChAccess','0','ModelPortBlock',{{struct('BlockId','','SignalId','')}})
  PROC_INT_BL1 - interrupt_pv : rtiproclib/PROC_INT_BL1  DSProperties=struct('RTI',struct('Version',uint32(4),'BlockType',struct('isSLSource',uint8(1),'isSLSink',uint8(0),'isHWSource',uint8(0),'isHWSink',uint8(0),'isSetup',uint8(1),'isInline',uint8(1),'isNonInline',uint8(0),'isInterrupt',uint8(0),'isChannelwise',uint8(0)),'IOBoardType','DSPROC','UnitType','','Identifier','INT','DialogType','ML','BlockSet','DSPROC','SlaveProcessor',''))  RTIBlockInterface=struct('OutputPortsActive',1,'OutputPortsWidth',int32(1),'OutputPortsName',{{'Interrupt'}},'FunctionCall',uint32(0),'DialogFcn','rtiprocintgui','InitLevel',3,'BlockDisplay',{{['Interrupt In 1\ninterrupt_pv \nBoard: 1'],'center'}},'IconTransparency','on','BlockName',struct('Token',{{'PROC_INT_BL1'}}))  RTIBlockParameters=struct('BoardNo',{{'1','OFF',[1 16]}},'ChannelNo',{{'1','OFF',[1 8]}},'AccessTyp',{{'Interrupt','OFF',[]}},'BinaryPoint',{{'0','OFF',[]}},'DataFormat',{{'unsigned','OFF',[]}},'BufferLength',{{'0','OFF',[]}},'MultiChAccess',{{'0','OFF',[]}},'ModelPortBlock',{{{struct('BlockId','','SignalId','')},'OFF',[]}})  RTISFcnParameters=struct('BoardNo','double','ChannelNo','double','AccessTyp','char','BinaryPoint','double','DataFormat','char','BufferLength','double')  RTIBlockParaDefault=struct('BoardNo','1','ChannelNo','1','AccessTyp','Interrupt','BinaryPoint','10','DataFormat','unsigned','BufferLength','0','MultiChAccess','0','ModelPortBlock',{{struct('BlockId','','SignalId','')}})
  PROC_INT_BL1 - interrupt_vsi : rtiproclib/PROC_INT_BL1  DSProperties=struct('RTI',struct('Version',uint32(4),'BlockType',struct('isSLSource',uint8(1),'isSLSink',uint8(0),'isHWSource',uint8(0),'isHWSink',uint8(0),'isSetup',uint8(1),'isInline',uint8(1),'isNonInline',uint8(0),'isInterrupt',uint8(0),'isChannelwise',uint8(0)),'IOBoardType','DSPROC','UnitType','','Identifier','INT','DialogType','ML','BlockSet','DSPROC','SlaveProcessor',''))  RTIBlockInterface=struct('OutputPortsActive',1,'OutputPortsWidth',int32(1),'OutputPortsName',{{'Interrupt'}},'FunctionCall',uint32(0),'DialogFcn','rtiprocintgui','InitLevel',3,'BlockDisplay',{{['Interrupt In 3\n interrupt_vsi\nBoard: 1'],'center'}},'IconTransparency','on','BlockName',struct('Token',{{'PROC_INT_BL1'}}))  RTIBlockParameters=struct('BoardNo',{{'1','OFF',[1 16]}},'ChannelNo',{{'3','OFF',[1 8]}},'AccessTyp',{{'Interrupt','OFF',[]}},'BinaryPoint',{{'0','OFF',[]}},'DataFormat',{{'unsigned','OFF',[]}},'BufferLength',{{'0','OFF',[]}},'MultiChAccess',{{'0','OFF',[]}},'ModelPortBlock',{{{struct('BlockId','','SignalId','')},'OFF',[]}})  RTISFcnParameters=struct('BoardNo','double','ChannelNo','double','AccessTyp','char','BinaryPoint','double','DataFormat','char','BufferLength','double')  RTIBlockParaDefault=struct('BoardNo','1','ChannelNo','1','AccessTyp','Interrupt','BinaryPoint','10','DataFormat','unsigned','BufferLength','0','MultiChAccess','0','ModelPortBlock',{{struct('BlockId','','SignalId','')}})
  PROC_SETUP_BL1 : rtiproclib/PROC_SETUP_BL1  DSProperties=struct('RTI',struct('Version',uint32(3),'BlockType',struct('isSLSource',uint8(0),'isSLSink',uint8(0),'isHWSource',uint8(0),'isHWSink',uint8(0),'isSetup',uint8(1),'isInline',uint8(1),'isNonInline',uint8(0),'isInterrupt',uint8(0),'isChannelwise',uint8(0)),'IOBoardType','DSPROC','UnitType','SETUP','Identifier','SETUP','DialogType','ML','BlockSet','NONE','SlaveProcessor',''))  RTIBlockInterface=struct('OutputPortsWidth',int32(0),'OutputPortsActive',0,'InitLevel',3,'DialogFcn','rtiprocsetupgui','BlockDisplay',{{['Processor Setup'],'auto'}},'IconTransparency','off','BlockName',struct('Token',{{'PROC_SETUP_BL1'}}))  RTIBlockParameters=struct('NumBoardsUsed',{{1,'OFF',[1 16]}},'ModelMode',{{1,'OFF',[]}},'IniFileList',{{struct('Fullname','','Filename','','Relname','','Assigned',0),'OFF',[]}},'SubsysList',{{struct('SharedAccess',1,'SetupBlockHandle',17122.000122070313,'SetupBlockName','FPGA_SETUP_BL1','SubsysName','fpga_dcmg','SubsysHandle',15989.000122070313,'SubsysPath','/fpga_dcmg','Assigned',1,'IniFilePath','D:\MarcosGomez\DCMG\dcmg_rtiFPGA/INI/fpga_dcmg_8403B8C1393193.ini','IniFileName','fpga_dcmg_8403B8C1393193','IniFileDate',739605.75260416663),'OFF',[]}},'AssignList',{{struct('BoardNumber',{1,2,3,4,5,6,7,8,9,10,11,12,13,14,15,16},'ModelType',{1,0,0,0,0,0,0,0,0,0,0,0,0,0,0,0},'ModelNo',{1,0,0,0,0,0,0,0,0,0,0,0,0,0,0,0},'ProgOption',{2,0,0,0,0,0,0,0,0,0,0,0,0,0,0,0},'IncludeBuild',{1,0,0,0,0,0,0,0,0,0,0,0,0,0,0,0},'IncludeProcAppl',{true,0,0,0,0,0,0,0,0,0,0,0,0,0,0,0}),'OFF',[]}},'ProcSetupHandles',{{-1,'OFF',[]}},'MaxNumBoards',{{16,'OFF',[]}},'ModelPath',{{'D:\MarcosGomez\DCMG','OFF',[]}},'FrameDir',{{[' '],'OFF',[]}},'TLCFileName',{{'rtiprocsetup','OFF',[]}},'IsNewBlock',{{0,'OFF',[]}},'NeedsCodeGen',{{0,'OFF',[]}})  RTISFcnParameters=struct('FrameDir','char','TLCFileName','char')  RTIBlockParaDefault=struct('NumBoardsUsed',1,'ModelMode',1,'IniFileList',struct('Fullname','','Filename','','Relname','','Assigned',''),'SubsysList',struct('SubsysName','','SubsysPath','','SubsysHandle','','SetupBlockHandle','','SetupBlockName','','Filename','','Relname','','IniFilePath','','IniFileName','','IniFileDate','','Assigned',''),'AssignList',struct('BoardNumber','','ModelType','','ModelNo','','ProgOption','','IncludeBuild','','IncludeProcAppl',''),'ProcSetupHandles',-1,'MaxNumBoards',16,'ModelPath',[' '],'FrameDir',[' '],'TLCFileName','rtiprocsetup','IsNewBlock',1,'NeedsCodeGen',0)
      settings: AttributesFormatString=FPGA-Build / Offline Simulation
  PROC_XDATA_WRITE_BL1 - d_bat : rtiproclib/PROC_XDATA_WRITE_BL1  DSProperties=struct('RTI',struct('Version',uint32(6),'BlockType',struct('isSLSource',uint8(0),'isSLSink',uint8(1),'isHWSource',uint8(0),'isHWSink',uint8(0),'isSetup',uint8(0),'isInline',uint8(1),'isNonInline',uint8(0),'isInterrupt',uint8(0),'isChannelwise',uint8(0)),'IOBoardType','DSPROC','UnitType','','Identifier','PHSWRITE','DialogType','ML','BlockSet','DSPROC','SlaveProcessor',''))  RTIBlockInterface=struct('InputPortsActive',true,'InputPortsWidth',{{'DYNAMICALLY_SIZED'}},'InputPortsDataType',{{'SS_DOUBLE'}},'InputPortsName',{{'Data'}},'InitLevel',3,'DialogFcn','rtiprocphswritegui','BlockDisplay',{{['Register Out 5\nd_bat\nGroup ID: 1 Board: 1'],'auto'}},'IconTransparency','on','BlockName',struct('Token',{{'PROC_XDATA_WRITE_BL1'}}))  RTIBlockParameters=struct('BoardNo',{{'1','OFF',[1 16]}},'ChannelNo',{{'5','OFF',[]}},'AccessTyp',{{'Register','OFF',[]}},'BinaryPoint',{{'0','OFF',[]}},'DataFormat',{{'unsigned','OFF',[]}},'BufferLength',{{'0','OFF',[]}},'GroupNo',{{'1','OFF',[]}},'MultiChAccess',{{'0','OFF',[]}},'InitOnly',{{'0','OFF',[]}},'InitValue',{{'0','OFF',[]}},'TLCFileName',{{'rtiprocphswrite','OFF',[]}},'ModelPortBlock',{{{struct('BlockId','','SignalId','')},'OFF',[]}})  RTISFcnParameters=struct('BoardNo','double','ChannelNo','double','GroupNo','double','AccessTyp','char','BinaryPoint','double','DataFormat','char','BufferLength','double','InitOnly','double','InitValue','double','TLCFileName','char')  RTIBlockParaDefault=struct('BoardNo','1','ChannelNo','0','AccessTyp','Register','BinaryPoint','10','DataFormat','signed','BufferLength','16','GroupNo','0','MultiChAccess','0','InitOnly','0','InitValue','0','TLCFileName','rtiprocphswrite','ModelPortBlock',{{struct('BlockId','','SignalId','','BusObject','')}})
  PROC_XDATA_WRITE_BL1 - d_pv : rtiproclib/PROC_XDATA_WRITE_BL1  DSProperties=struct('RTI',struct('Version',uint32(6),'BlockType',struct('isSLSource',uint8(0),'isSLSink',uint8(1),'isHWSource',uint8(0),'isHWSink',uint8(0),'isSetup',uint8(0),'isInline',uint8(1),'isNonInline',uint8(0),'isInterrupt',uint8(0),'isChannelwise',uint8(0)),'IOBoardType','DSPROC','UnitType','','Identifier','PHSWRITE','DialogType','ML','BlockSet','DSPROC','SlaveProcessor',''))  RTIBlockInterface=struct('InputPortsActive',true,'InputPortsWidth',{{'DYNAMICALLY_SIZED'}},'InputPortsDataType',{{'SS_DOUBLE'}},'InputPortsName',{{'Data'}},'InitLevel',3,'DialogFcn','rtiprocphswritegui','BlockDisplay',{{['Register Out 4\nd_pv\nGroup ID: 1 Board: 1'],'auto'}},'IconTransparency','on','BlockName',struct('Token',{{'PROC_XDATA_WRITE_BL1'}}))  RTIBlockParameters=struct('BoardNo',{{'1','OFF',[1 16]}},'ChannelNo',{{'4','OFF',[]}},'AccessTyp',{{'Register','OFF',[]}},'BinaryPoint',{{'0','OFF',[]}},'DataFormat',{{'unsigned','OFF',[]}},'BufferLength',{{'0','OFF',[]}},'GroupNo',{{'1','OFF',[]}},'MultiChAccess',{{'0','OFF',[]}},'InitOnly',{{'0','OFF',[]}},'InitValue',{{'0','OFF',[]}},'TLCFileName',{{'rtiprocphswrite','OFF',[]}},'ModelPortBlock',{{{struct('BlockId','','SignalId','')},'OFF',[]}})  RTISFcnParameters=struct('BoardNo','double','ChannelNo','double','GroupNo','double','AccessTyp','char','BinaryPoint','double','DataFormat','char','BufferLength','double','InitOnly','double','InitValue','double','TLCFileName','char')  RTIBlockParaDefault=struct('BoardNo','1','ChannelNo','0','AccessTyp','Register','BinaryPoint','10','DataFormat','signed','BufferLength','16','GroupNo','0','MultiChAccess','0','InitOnly','0','InitValue','0','TLCFileName','rtiprocphswrite','ModelPortBlock',{{struct('BlockId','','SignalId','','BusObject','')}})
  PROC_XDATA_WRITE_BL1 - da : rtiproclib/PROC_XDATA_WRITE_BL1  DSProperties=struct('RTI',struct('Version',uint32(6),'BlockType',struct('isSLSource',uint8(0),'isSLSink',uint8(1),'isHWSource',uint8(0),'isHWSink',uint8(0),'isSetup',uint8(0),'isInline',uint8(1),'isNonInline',uint8(0),'isInterrupt',uint8(0),'isChannelwise',uint8(0)),'IOBoardType','DSPROC','UnitType','','Identifier','PHSWRITE','DialogType','ML','BlockSet','DSPROC','SlaveProcessor',''))  RTIBlockInterface=struct('InputPortsActive',true,'InputPortsWidth',{{'DYNAMICALLY_SIZED'}},'InputPortsDataType',{{'SS_DOUBLE'}},'InputPortsName',{{'Data'}},'InitLevel',3,'DialogFcn','rtiprocphswritegui','BlockDisplay',{{['Register Out 1\nda \nGroup ID: 1 Board: 1'],'auto'}},'IconTransparency','on','BlockName',struct('Token',{{'PROC_XDATA_WRITE_BL1'}}))  RTIBlockParameters=struct('BoardNo',{{'1','OFF',[1 16]}},'ChannelNo',{{'1','OFF',[]}},'AccessTyp',{{'Register','OFF',[]}},'BinaryPoint',{{'0','OFF',[]}},'DataFormat',{{'unsigned','OFF',[]}},'BufferLength',{{'0','OFF',[]}},'GroupNo',{{'1','OFF',[]}},'MultiChAccess',{{'0','OFF',[]}},'InitOnly',{{'0','OFF',[]}},'InitValue',{{'0','OFF',[]}},'TLCFileName',{{'rtiprocphswrite','OFF',[]}},'ModelPortBlock',{{{struct('BlockId','','SignalId','')},'OFF',[]}})  RTISFcnParameters=struct('BoardNo','double','ChannelNo','double','GroupNo','double','AccessTyp','char','BinaryPoint','double','DataFormat','char','BufferLength','double','InitOnly','double','InitValue','double','TLCFileName','char')  RTIBlockParaDefault=struct('BoardNo','1','ChannelNo','0','AccessTyp','Register','BinaryPoint','10','DataFormat','signed','BufferLength','16','GroupNo','0','MultiChAccess','0','InitOnly','0','InitValue','0','TLCFileName','rtiprocphswrite','ModelPortBlock',{{struct('BlockId','','SignalId','','BusObject','')}})
  PROC_XDATA_WRITE_BL1 - db : rtiproclib/PROC_XDATA_WRITE_BL1  DSProperties=struct('RTI',struct('Version',uint32(6),'BlockType',struct('isSLSource',uint8(0),'isSLSink',uint8(1),'isHWSource',uint8(0),'isHWSink',uint8(0),'isSetup',uint8(0),'isInline',uint8(1),'isNonInline',uint8(0),'isInterrupt',uint8(0),'isChannelwise',uint8(0)),'IOBoardType','DSPROC','UnitType','','Identifier','PHSWRITE','DialogType','ML','BlockSet','DSPROC','SlaveProcessor',''))  RTIBlockInterface=struct('InputPortsActive',true,'InputPortsWidth',{{'DYNAMICALLY_SIZED'}},'InputPortsDataType',{{'SS_DOUBLE'}},'InputPortsName',{{'Data'}},'InitLevel',3,'DialogFcn','rtiprocphswritegui','BlockDisplay',{{['Register Out 2\ndb\nGroup ID: 1 Board: 1'],'auto'}},'IconTransparency','on','BlockName',struct('Token',{{'PROC_XDATA_WRITE_BL1'}}))  RTIBlockParameters=struct('BoardNo',{{'1','OFF',[1 16]}},'ChannelNo',{{'2','OFF',[]}},'AccessTyp',{{'Register','OFF',[]}},'BinaryPoint',{{'0','OFF',[]}},'DataFormat',{{'unsigned','OFF',[]}},'BufferLength',{{'0','OFF',[]}},'GroupNo',{{'1','OFF',[]}},'MultiChAccess',{{'0','OFF',[]}},'InitOnly',{{'0','OFF',[]}},'InitValue',{{'0','OFF',[]}},'TLCFileName',{{'rtiprocphswrite','OFF',[]}},'ModelPortBlock',{{{struct('BlockId','','SignalId','')},'OFF',[]}})  RTISFcnParameters=struct('BoardNo','double','ChannelNo','double','GroupNo','double','AccessTyp','char','BinaryPoint','double','DataFormat','char','BufferLength','double','InitOnly','double','InitValue','double','TLCFileName','char')  RTIBlockParaDefault=struct('BoardNo','1','ChannelNo','0','AccessTyp','Register','BinaryPoint','10','DataFormat','signed','BufferLength','16','GroupNo','0','MultiChAccess','0','InitOnly','0','InitValue','0','TLCFileName','rtiprocphswrite','ModelPortBlock',{{struct('BlockId','','SignalId','','BusObject','')}})
  PROC_XDATA_WRITE_BL1 - dc : rtiproclib/PROC_XDATA_WRITE_BL1  DSProperties=struct('RTI',struct('Version',uint32(6),'BlockType',struct('isSLSource',uint8(0),'isSLSink',uint8(1),'isHWSource',uint8(0),'isHWSink',uint8(0),'isSetup',uint8(0),'isInline',uint8(1),'isNonInline',uint8(0),'isInterrupt',uint8(0),'isChannelwise',uint8(0)),'IOBoardType','DSPROC','UnitType','','Identifier','PHSWRITE','DialogType','ML','BlockSet','DSPROC','SlaveProcessor',''))  RTIBlockInterface=struct('InputPortsActive',true,'InputPortsWidth',{{'DYNAMICALLY_SIZED'}},'InputPortsDataType',{{'SS_DOUBLE'}},'InputPortsName',{{'Data'}},'InitLevel',3,'DialogFcn','rtiprocphswritegui','BlockDisplay',{{['Register Out 3\ndc\nGroup ID: 1 Board: 1'],'auto'}},'IconTransparency','on','BlockName',struct('Token',{{'PROC_XDATA_WRITE_BL1'}}))  RTIBlockParameters=struct('BoardNo',{{'1','OFF',[1 16]}},'ChannelNo',{{'3','OFF',[]}},'AccessTyp',{{'Register','OFF',[]}},'BinaryPoint',{{'0','OFF',[]}},'DataFormat',{{'unsigned','OFF',[]}},'BufferLength',{{'0','OFF',[]}},'GroupNo',{{'1','OFF',[]}},'MultiChAccess',{{'0','OFF',[]}},'InitOnly',{{'0','OFF',[]}},'InitValue',{{'0','OFF',[]}},'TLCFileName',{{'rtiprocphswrite','OFF',[]}},'ModelPortBlock',{{{struct('BlockId','','SignalId','')},'OFF',[]}})  RTISFcnParameters=struct('BoardNo','double','ChannelNo','double','GroupNo','double','AccessTyp','char','BinaryPoint','double','DataFormat','char','BufferLength','double','InitOnly','double','InitValue','double','TLCFileName','char')  RTIBlockParaDefault=struct('BoardNo','1','ChannelNo','0','AccessTyp','Register','BinaryPoint','10','DataFormat','signed','BufferLength','16','GroupNo','0','MultiChAccess','0','InitOnly','0','InitValue','0','TLCFileName','rtiprocphswrite','ModelPortBlock',{{struct('BlockId','','SignalId','','BusObject','')}})
  RTI Data : Subsystem  Tag=struct('RTIDataServer',struct('RTIDataServerVs','2','RTIModelDescription','struct(''main'',''dcmg'',''sub'','''',''isMp'',0)'))  LoadFcn="if exist('rtidc'), try,  rtidc('DataHostBlockClbLoad', gcbh); catch, disp(['Warning: ''LoadFcn'' for RTI Data block failed: ' lasterr]); end, end,"  mask(RTI_DATA_HOST){}
      mask help:
      | RTI Data Block.
      | This block is used by RTI to store internal model-dependent data.
      | Please keep this block on the root level of the model. Deleting this block will result in data loss.
      |
      | NEVER DELETE OR COPY THIS BLOCK!
      settings: CopyFcn="if exist('rtidc'), try,  rtidc('DataHostBlockClbCopy', gcbh); catch, disp(['Warning: ''CopyFcn'' for RTI Data block failed: ' lasterr]); end, end,"  DeleteFcn="if exist('rtidc'), try,  rtidc('DataHostBlockClbDelete', gcbh); catch, disp(['Warning: ''DeleteFcn'' for RTI Data block failed: ' lasterr]); end, end,"  ModelCloseFcn="if exist('rtidc'), try,  rtidc('DataHostBlockClbModelClose', gcbh); catch, disp(['Warning: ''ModelCloseFcn'' for RTI Data block failed: ' lasterr]); end, end,"  PreSaveFcn="if exist('rtidc'), try,  rtidc('DataHostBlockClbPreSave', gcbh); catch, disp(['Warning: ''PreSaveFcn'' for RTI Data block failed: ' lasterr]); end, end,"  PostSaveFcn="if exist('rtidc'), try,  rtidc('DataHostBlockClbPostSave', gcbh); catch, disp(['Warning: ''PostSaveFcn'' for RTI Data block failed: ' lasterr]); end, end,"  NameChangeFcn="if exist('rtidc'), try,  rtidc('DataHostBlockClbNameChange', gcbh); catch, disp(['Warning: ''NameChangeFcn'' for RTI Data block failed: ' lasterr]); end, end,"
      mask Help:
      | RTI Data Block.
      | This block is used by RTI to store internal model-dependent data.
      | Please keep this block on the root level of the model. Deleting this block will result in data loss.
      | 
      | NEVER DELETE OR COPY THIS BLOCK!
      mask Display:
      | text(0.5, 0.5, 'RTI Data', 'HorizontalAlignment', 'center');
      | plot([1 0]);
  Rate Transition{,1..3,8..10} (7 alike) : RateTransition  Deterministic=off
  Rate Transition{4..7} (4 alike) : RateTransition  Deterministic=off  OutPortSampleTimeOpt=Inherit
  Subsystem : Subsystem
  Subsystem1 : Subsystem
  Sum{,1..11} (12 alike) : Sum  Inputs=|++
  da : Constant
  db : Constant  Value=0
  dc : Constant  Value=0.5
  fixedgain_i : Gain  Gain=fixedgain_i
  fixedgain_i1 : Gain  Gain=fixedgain_i
  fixedgain_i2 : Gain  Gain=fixedgain_i
  fixedgain_ibat : Gain  Gain=fixedgain_ibat
  fixedgain_ioavsi : Gain  Gain=fixedgain_i
  fixedgain_iobvsi : Gain  Gain=fixedgain_i
  fixedgain_ipv : Gain  Gain=fixedgain_ipv
  fixedgain_vavsi : Gain  Gain=fixedgain_v
  fixedgain_vbvsi : Gain  Gain=200*10
  fixedgain_vcvsi : Gain  Gain=fixedgain_v
  fixedgain_vdc : Gain  Gain=fixedgain_vdc
  fixedgain_vpv : Gain  Gain=fixedgain_vpv
  fpga_dcmg : Subsystem
  gain_iavsi : Gain  Gain=gain_iavsi
  gain_ibat : Gain  Gain=gain_ibat
  gain_ibvsi : Gain  Gain=gain_ibvsi
  gain_icvsi : Gain  Gain=gain_icvsi
  gain_ioavsi : Gain  Gain=gain_ioavsi
  gain_iobvsi : Gain  Gain=gain_iobvsi
  gain_ipv : Gain  Gain=gain_ipv
  gain_vavsi : Gain  Gain=gain_vavsi
  gain_vbvsi : Gain  Gain=gain_vbvsi
  gain_vcvsi : Gain  Gain=gain_vcvsi
  gain_vdc : Gain  Gain=gain_vdc
  gain_vpv : Gain  Gain=gain_vpv
  iocvsi : Sum  Inputs=-|-
  offset_iavsi : Constant  Value=offset_iavsi
  offset_ibat : Constant  Value=offset_ibat
  offset_ibvsi : Constant  Value=offset_ibvsi
  offset_icvsi : Constant  Value=offset_icvsi
  offset_ioavsi : Constant  Value=offset_ioavsi
  offset_iobvsi : Constant  Value=offset_iobvsi
  offset_ipv : Constant  Value=offset_ipv
  offset_vavsi : Constant  Value=offset_vavsi
  offset_vbvsi : Constant  Value=offset_vbvsi
  offset_vcvsi : Constant  Value=offset_vcvsi
  offset_vdc : Constant  Value=offset_vdc
  offset_vpv : Constant  Value=offset_vpv
  wires:
  Subsystem1/3(Out3) -> Rate Transition3/1
  Subsystem1/1(Out1) -> Rate Transition1/1
  Subsystem1/2(Out2) -> Rate Transition2/1
  PROC_INT_BL1 - interrupt_vsi/1 -> Subsystem1/Trigger
  Constant/1 -> Integrator/1
  Integrator/1 -> Rate Transition/1
  Rate Transition/1 -> Subsystem1/1(In1)
  Rate Transition1/1 -> Gain/1
  Rate Transition2/1 -> Gain1/1
  Rate Transition3/1 -> Gain2/1
  fixedgain_i/1 -> Sum2/1
  offset_iavsi/1 -> Sum2/2
  Sum2/1 -> gain_iavsi/1
  ADC_CLASS1_BL1/1 -> fixedgain_i/1
  fixedgain_i1/1 -> Sum3/1
  Sum3/1 -> gain_ibvsi/1
  offset_ibvsi/1 -> Sum3/2
  ADC_CLASS1_BL2/1 -> fixedgain_i1/1
  fixedgain_i2/1 -> Sum4/1
  Sum4/1 -> gain_icvsi/1
  offset_icvsi/1 -> Sum4/2
  ADC_CLASS1_BL3/1 -> fixedgain_i2/1
  gain_icvsi/1 -> ?
  gain_ibvsi/1 -> ?
  gain_iavsi/1 -> ?
  Discrete Transfer Fcn2/1 -> Rate Transition7/1, Rate Transition8/1
  Rate Transition5/1 -> MPPT_system/1(v_PV)
  Rate Transition6/1 -> MPPT_system/2(i_PV)
  Discrete Transfer Fcn1/1 -> Rate Transition6/1
  fixedgain_vpv/1 -> Sum5/1
  Discrete Transfer Fcn/1 -> Rate Transition5/1
  ADC_CLASS1_BL6/1 -> fixedgain_ipv/1
  ADC_CLASS1_BL7/1 -> fixedgain_vpv/1
  fixedgain_vdc/1 -> Sum/1
  gain_ipv/1 -> Discrete Transfer Fcn1/1
  Sum6/1 -> gain_ipv/1
  gain_vpv/1 -> Discrete Transfer Fcn/1
  Sum/1 -> gain_vdc/1
  offset_vdc/1 -> Sum/2
  offset_vpv/1 -> Sum5/2
  fixedgain_ipv/1 -> Sum6/1
  gain_vdc/1 -> Discrete Transfer Fcn2/1
  Rate Transition4/1 -> PROC_XDATA_WRITE_BL1 - d_pv/1
  offset_ipv/1 -> Sum6/2
  Rate Transition7/1 -> MPPT_system/3(v_DC)
  Sum5/1 -> gain_vpv/1
  MPPT_system/1(d) -> Rate Transition4/1
  PROC_INT_BL1 - interrupt_pv/1 -> MPPT_system/Trigger
  ADC_CLASS1_BL5/1 -> fixedgain_vdc/1
  gain_ibat/1 -> Rate Transition9/1
  Subsystem/1(y1) -> Rate Transition10/1
  offset_ibat/1 -> Sum8/2
  Rate Transition8/1 -> Subsystem/1(v_dc)
  PROC_INT_BL1 - interrupt_bat/1 -> Subsystem/Trigger
  Sum8/1 -> gain_ibat/1
  Gain3/1 -> PROC_XDATA_WRITE_BL1 - d_bat/1
  Rate Transition9/1 -> Subsystem/2(i_bat)
  fixedgain_ibat/1 -> Sum8/1
  ADC_CLASS1_BL9/1 -> fixedgain_ibat/1
  Gain/1 -> PROC_XDATA_WRITE_BL1 - da/1
  Gain1/1 -> PROC_XDATA_WRITE_BL1 - db/1
  Gain2/1 -> PROC_XDATA_WRITE_BL1 - dc/1
  Sum9/1 -> gain_vcvsi/1
  fixedgain_vbvsi/1 -> Sum7/1
  fixedgain_vavsi/1 -> Sum1/1
  fixedgain_vcvsi/1 -> Sum9/1
  offset_vavsi/1 -> Sum1/2
  offset_vbvsi/1 -> Sum7/2
  Sum1/1 -> gain_vavsi/1
  ADC_CLASS1_BL10/1 -> fixedgain_vcvsi/1
  Sum7/1 -> gain_vbvsi/1
  ADC_CLASS1_BL4/1 -> fixedgain_vavsi/1
  offset_vcvsi/1 -> Sum9/2
  ADC_CLASS1_BL8/1 -> fixedgain_vbvsi/1
  gain_iobvsi/1 -> iocvsi/2
  fixedgain_ioavsi/1 -> Sum10/1
  fixedgain_iobvsi/1 -> Sum11/1
  offset_ioavsi/1 -> Sum10/2
  gain_ioavsi/1 -> iocvsi/1
  offset_iobvsi/1 -> Sum11/2
  Sum10/1 -> gain_ioavsi/1
  Sum11/1 -> gain_iobvsi/1
  ADC_CLASS2_BL1/1 -> fixedgain_ioavsi/1
  ADC_CLASS2_BL2/1 -> fixedgain_iobvsi/1
  iocvsi/1 -> ?
  db/1 -> ?
  da/1 -> ?
  dc/1 -> ?
  Rate Transition10/1 -> Gain3/1
